simulink model "Sim2"  (R2019b)
settings: Solver=VariableStepAuto  StartTime=0.0  StopTime=10.0  RelTol=1e-3
values from neighbouring files (symbols this model uses):
  A = [[-.0714 0];[1 0]]    [DC_Motor_Analysis.m]    (also in Part1.m = [[A11 A12];[A21 A22]]; SS_lab.m = [-2.6788 0;1 0]; mathModel.mat = [-2.28310502283  0; 1  0])
  B = [3.40786 0].'    [DC_Motor_Analysis.m]    (also in Part1.m = [B1 B2].'; SS_lab.m = [12.05465;0]; mathModel.mat = [103.062962083 0])
  feedForwardGain = 1/dcGain    [DC_Motor_Analysis.m]
  K = [k1 k2]    [DC_Motor_Analysis.m]    (also in Part3.m = double(linsolve(meatMat, potatoesMat)))
settings Model: Creator=justinf  LastModifiedBy=justinf

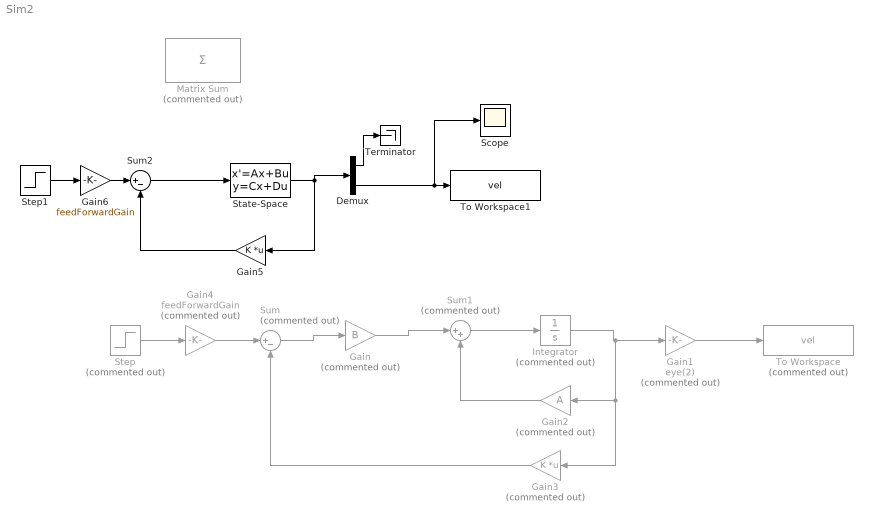
== system Sim2 ==
  Demux : Demux  Outputs=2
  Gain : Gain  Commented=on  Gain=B
  Gain1 : Gain  Commented=on  Gain=eye(2)
  Gain2 : Gain  Commented=on  Gain=A
  Gain3 : Gain  Commented=on  Gain=K  Multiplication=Matrix(K*u)
  Gain4 : Gain  Commented=on  Gain=feedForwardGain
  Gain5 : Gain  Gain=K  Multiplication=Matrix(K*u)
  Gain6 : Gain  Gain=feedForwardGain
  Integrator : Integrator  Commented=on
  Matrix Sum : Sum  Commented=on  Inputs=+
  Scope : Scope
  State-Space : StateSpace  A=A  B=B  C=eye(2)  D=[0;0]  InitialCondition=0
  Step : Step  Commented=on  SampleTime=0
  Step1 : Step  Time=0  SampleTime=0
  Sum : Sum  Commented=on  Inputs=|+-
  Sum1 : Sum  Commented=on  Inputs=|++
  Sum2 : Sum  Inputs=|+-
  Terminator : Terminator
  To Workspace : ToWorkspace  Commented=on  VariableName=vel  SaveFormat=Timeseries  SampleTime=-1
  To Workspace1 : ToWorkspace  VariableName=vel  SampleTime=-1
  wires:
  Step/1 -> Gain4/1
  Gain/1 -> Sum1/1
  Sum1/1 -> Integrator/1
  Integrator/1 -> Gain3/1, Gain2/1, Gain1/1
  Gain2/1 -> Sum1/2
  Gain3/1 -> Sum/2
  Sum/1 -> Gain/1
  Gain1/1 -> To Workspace/1
  Gain4/1 -> Sum/1
  Step1/1 -> Gain6/1
  Gain6/1 -> Sum2/1
  Sum2/1 -> State-Space/1
  Gain5/1 -> Sum2/2
  State-Space/1 -> Gain5/1, Demux/1
  Demux/1 -> Terminator/1
  Demux/2 -> Scope/1, To Workspace1/1
